simulink model "experiment_1_lab_05"  (Simulink 7.1)
settings: Solver=ode45  StartTime=0.0  StopTime=10.0  RelTol=1e-3
InitFcn:
  | R1=2;
  | R2=4;
  | L1=0.5;
  | L2=1;
  | C=3/8;
settings Model: Creator=ALUNO  LastModifiedBy=ALUNO

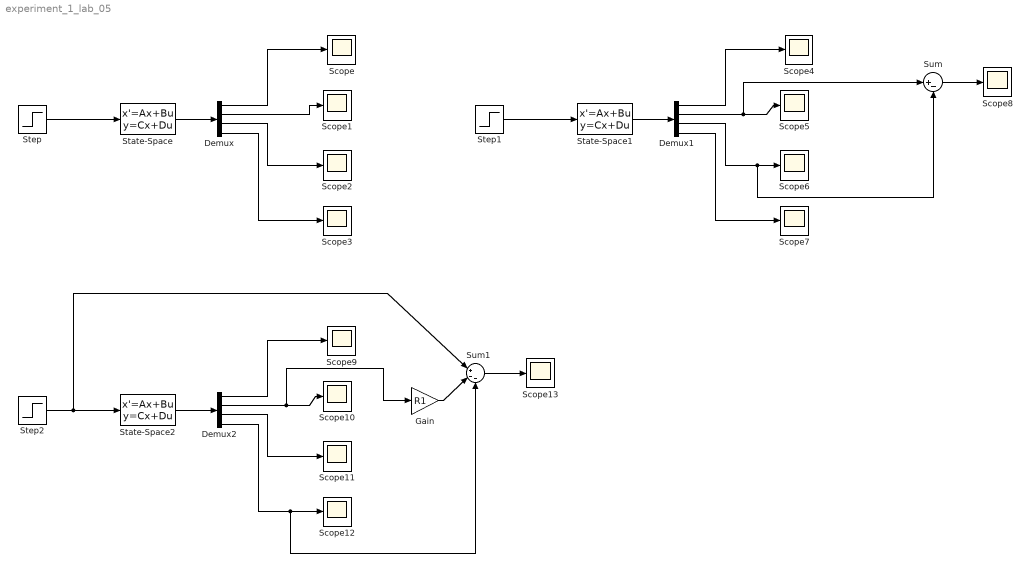
== system experiment_1_lab_05 ==
  Demux : Demux
  Demux1 : Demux
  Demux2 : Demux
  Gain : Gain  Gain=R1  ParameterDataType=sfix(16)  ParameterScaling=2^0  OutDataType=sfix(16)  OutScaling=2^0
  Scope{,1..13} (14 alike) : Scope
      Scope10 settings: SaveName=ScopeData9
      Scope11 settings: SaveName=ScopeData10
      Scope12 settings: SaveName=ScopeData11
      Scope13 settings: SaveName=ScopeData12
      Scope2 settings: SaveName=ScopeData2
      Scope3 settings: SaveName=ScopeData3
      Scope4 settings: SaveName=ScopeData4
      Scope5 settings: SaveName=ScopeData5
      Scope6 settings: SaveName=ScopeData6
      Scope7 settings: SaveName=ScopeData7
      Scope8 settings: SaveName=ScopeData8
      Scope9 settings: SaveName=ScopeData13
  State-Space : StateSpace  A=[-R1/L1,0,-1/L1;0,-R2/L2,1/L2;1/C,-1/C,0]  B=[1/L1;0;0]  C=[0,R2,0;1,0,0;0,1,0;0,0,1]  D=[0;0;0;0]
  State-Space1 : StateSpace  A=[-R1/L1,0,-1/L1;0,-R2/L2,1/L2;1/C,-1/C,0]  B=[1/L1;0;0]  C=[0,R2,0;1,0,0;0,1,0;0,0,1]  D=[0;0;0;0]
  State-Space2 : StateSpace  A=[-R1/L1,0,-1/L1;0,-R2/L2,1/L2;1/C,-1/C,0]  B=[1/L1;0;0]  C=[0,R2,0;1,0,0;0,1,0;0,0,1]  D=[0;0;0;0]
  Step : Step  Time=0  SampleTime=0
  Step1 : Step  Time=0  SampleTime=0
  Step2 : Step  Time=0  SampleTime=0
  Sum : Sum  Inputs=|+-  OutDataType=sfix(16)  OutScaling=2^0
  Sum1 : Sum  Inputs=|+--  OutDataType=sfix(16)  OutScaling=2^0
  wires:
  Step/1 -> State-Space/1
  State-Space/1 -> Demux/1
  Demux/1 -> Scope/1
  Demux/2 -> Scope1/1
  Demux/3 -> Scope2/1
  Demux/4 -> Scope3/1
  Step1/1 -> State-Space1/1
  State-Space1/1 -> Demux1/1
  Demux1/1 -> Scope4/1
  Demux1/2 -> Scope5/1, Sum/1
  Demux1/3 -> Scope6/1, Sum/2
  Demux1/4 -> Scope7/1
  Sum/1 -> Scope8/1
  Step2/1 -> State-Space2/1, Sum1/1
  State-Space2/1 -> Demux2/1
  Demux2/1 -> Scope9/1
  Demux2/2 -> Scope10/1, Gain/1
  Demux2/3 -> Scope11/1
  Demux2/4 -> Scope12/1, Sum1/3
  Sum1/1 -> Scope13/1
  Gain/1 -> Sum1/2
